simulink model "EulerEqs"  (R2020b)
settings: Solver=FixedStepAuto  StartTime=0.0  StopTime=200  FixedStep=sim_constants.time_step  RelTol=1E-6  AbsTol=1E-4
undefined symbols (not defined in the file or in its folder): sim_constants
libraries: vrlib x1
settings Model: Creator=newpo  LastModifiedBy=valerie

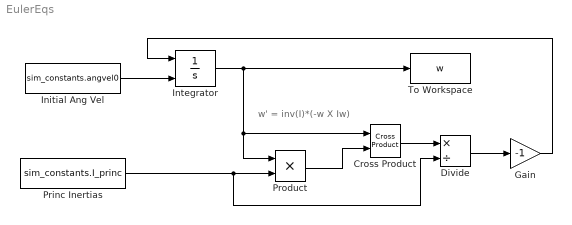
== system EulerEqs ==
  note: w' = inv(I)*(-w X Iw)
  Cross Product : vrlib/Utilities/Cross Product
  Divide : Product  Inputs=*/
  Gain : Gain  Gain=-1
  Initial Ang Vel : Constant  Value=sim_constants.angvel0
  Integrator : Integrator  InitialConditionSource=external
  Princ Inertias : Constant  Value=sim_constants.I_princ
  Product : Product
  To Workspace : ToWorkspace  VariableName=w  SampleTime=-1
  wires:
  Integrator/1 -> Cross Product/1, Product/1, To Workspace/1
  Gain/1 -> Integrator/1
  Cross Product/1 -> Divide/1
  Princ Inertias/1 -> Product/2, Divide/2
  Product/1 -> Cross Product/2
  Divide/1 -> Gain/1
  Initial Ang Vel/1 -> Integrator/2
